simulink model "SistemaUrinarioMasculino"  (R2024b)
settings: Solver=VariableStepAuto  StartTime=0.0  StopTime=30  RelTol=1e-3
libraries: slpidlib x1
settings DataIOCC: ReturnWorkspaceOutputs=off  TimeSaveName=t
settings DebuggingCC: AlgebraicLoopMsg=none  ArtificialAlgebraicLoopMsg=none

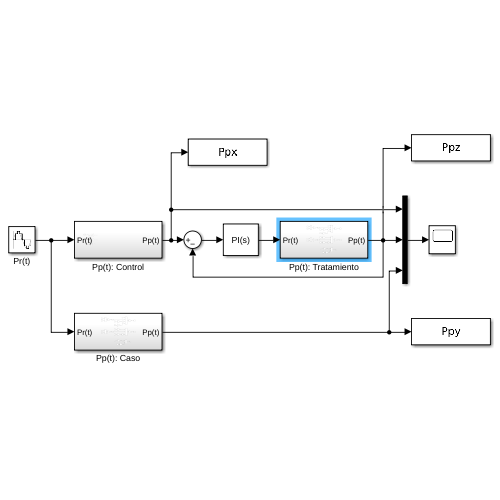
[thumbnail: Simulink's stored preview of the top-level diagram]
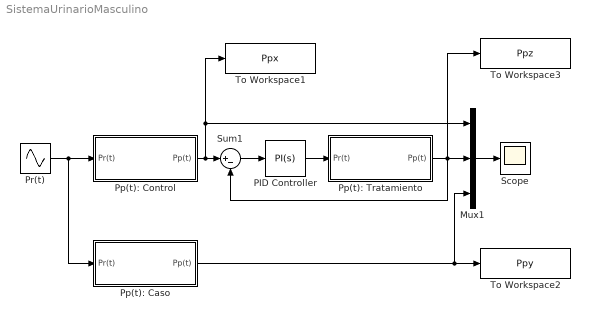
== system SistemaUrinarioMasculino ==
  Mux1 : Mux  Inputs=3
  PID Controller : slpidlib/PID Controller  Controller=PI  Form=Parallel  TimeDomain=Continuous-time  UseExternalTs=off  SampleTime=-1  IntegratorMethod=Forward Euler  FilterMethod=Forward Euler  ControllerParametersSource=internal  P=0.0233322963423837  I=449.984445135772  UseKiTs=off  D=0  UseExternalDerivativeSource=off  N=100  UseFilter=on  TunerSelectOption=Transfer Function Based (PID Tuner App)  InitialConditionSource=internal  InitialConditionForIntegrator=0  InitialConditionForFilter=0  DifferentiatorICPrevScaledInput=0  ExternalReset=none  TrackingMode=off  Kt=1  LimitOutput=off  SatLimitsSource=internal  UpperSaturationLimit=inf  LowerSaturationLimit=-inf  LinearizeAsGain=on  AntiWindupMode=none  Kb=1  LimitIntegrator=off  UpperIntegratorSaturationLimit=inf  LowerIntegratorSaturationLimit=-inf  POutMin=[]  POutMax=[]  IOutMin=[]  IOutMax=[]  DOutMin=[]  DOutMax=[]  NOutMin=[]  NOutMax=[]  SumOutMin=[]  SumOutMax=[]  SaturationOutMin=[]  SaturationOutMax=[]  PParamMin=[]  PParamMax=[]  IParamMin=[]  IParamMax=[]  DParamMin=[]  DParamMax=[]  NParamMin=[]  NParamMax=[]  KbParamMin=[]  KbParamMax=[]  KtParamMin=[]  KtParamMax=[]  KbOutMin=[]  KbOutMax=[]  KtOutMin=[]  KtOutMax=[]  IntegratorOutMin=[]  IntegratorOutMax=[]  FilterOutMin=[]  FilterOutMax=[]  SumI1OutMin=[]  SumI1OutMax=[]  SumI2OutMin=[]  SumI2OutMax=[]  SumI3OutMin=[]  SumI3OutMax=[]  SumI4OutMin=[]  SumI4OutMax=[]  SumDOutMin=[]  SumDOutMax=[]  DifferentiatorOutMin=[]  DifferentiatorOutMax=[]  FilterDiffOutCoefMin=[]  FilterDiffOutCoefMax=[]  ReciprocalOutMin=[]  ReciprocalOutMax=[]  SumDenOutMin=[]  SumDenOutMax=[]  SumNumOutMin=[]  SumNumOutMax=[]  DivideOutMin=[]  DivideOutMax=[]  UdiffTsProdOutMin=[]  UdiffTsProdOutMax=[]  NTsProdOutMin=[]  NTsProdOutMax=[]  UintegralTsProdOutMin=[]  UintegralTsProdOutMax=[]  UngainTsProdOutMin=[]  UngainTsProdOutMax=[]  ClampingZeroOutDataTypeStr=Inherit: Inherit via back propagation  ClampingZeroOutMin=[]  ClampingZeroOutMax=[]  FilterDenConstantOutDataTypeStr=Inherit: Inherit via back propagation  FilterDenConstantOutMin=[]  FilterDenConstantOutMax=[]  PCopyOutDataTypeStr=Inherit: Inherit via back propagation  PCopyOutMin=[]  PCopyOutMax=[]  NCopyOutDataTypeStr=Inherit: Inherit via back propagation  NCopyOutMin=[]  NCopyOutMax=[]  IntegratorContinuousStateAttributes=''  IntegratorStateMustResolveToSignalObject=off  IntegratorRTWStateStorageClass=Auto  FilterContinuousStateAttributes=''  FilterStateMustResolveToSignalObject=off  FilterRTWStateStorageClass=Auto  ParallelPVariant=InternalParameters  IdealPVariant=Disabled  IVariant=InternalParameters  DVariant=Disabled  IntegratorVariant=Continuous  SatVariant=Disabled  AWVariant=Passthrough  PCopyVariant=Disabled  TRVariant=Disabled  FdbkBlocksVariant=Forward  IdealPFdbkVariant=Disabled  SatFdbkVariant=Disabled  DerivativeFilterVariant=Disabled  NVariant=Disabled  NCopyVariant=Disabled_SignalSpec  FilterICVariant=Disabled  IntegratorICVariant=InternalICs  ExternalResetVariant=Disabled  TRSumVariant=Passthrough  SumFdbkVariant=Disabled  SumVariant=Sum_PI  TsampFilterVariant=InternalTs  TsampNgainVariant=Passthrough  TsampIntegralVariant=Disabled_SignalSpec  ExternalSaturationOutDataTypeStr=Inherit: Same as second input  DerivativeSourceVariant=Disabled  PreIntVariant=InternalPreInt
  Pp(t): Caso : Subsystem
  Pp(t): Control : Subsystem
  Pp(t): Tratamiento : Subsystem
  Pr(t) : Sin  Frequency=1.5708  SampleTime=0.001
  Scope : Scope
  Sum1 : Sum  Inputs=|+-
  To Workspace1 : ToWorkspace  VariableName=Ppx  SampleTime=-1
  To Workspace2 : ToWorkspace  VariableName=Ppy  SampleTime=-1
  To Workspace3 : ToWorkspace  VariableName=Ppz  SampleTime=-1
  wires:
  Pr(t)/1 -> Pp(t): Caso/1(Pr(t)), Pp(t): Control/1(Pr(t))
  Pp(t): Control/1(Pp(t)) -> Mux1/1, To Workspace1/1, Sum1/1
  Sum1/1 -> PID Controller/1
  Pp(t): Caso/1(Pp(t)) -> Mux1/3, To Workspace2/1
  PID Controller/1 -> Pp(t): Tratamiento/1(Pr(t))
  Pp(t): Tratamiento/1(Pp(t)) -> Sum1/2, To Workspace3/1, Mux1/2
  Mux1/1 -> Scope/1

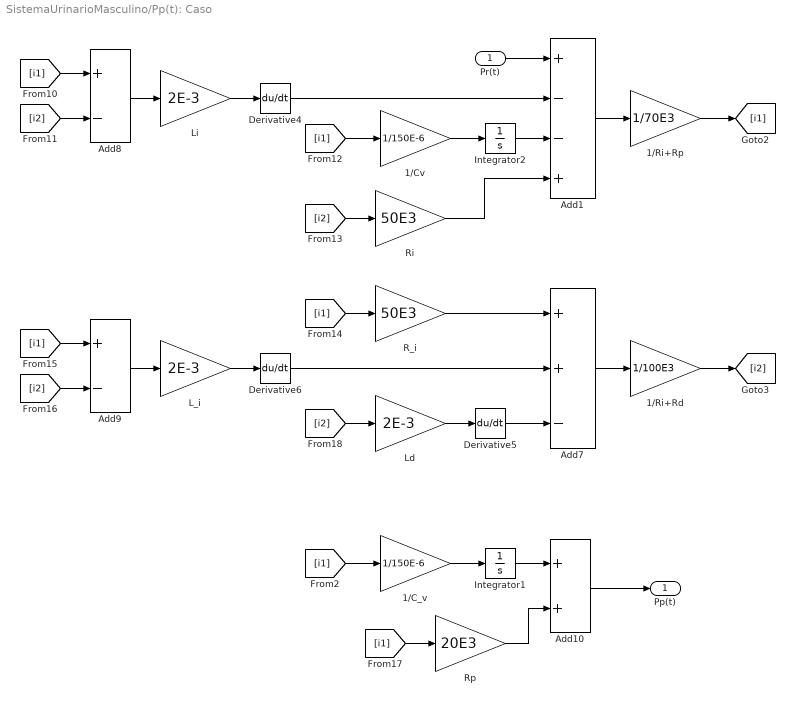
== system SistemaUrinarioMasculino/Pp(t): Caso ==
  Pr(t) : Inport
  1/C_v : Gain  Gain=1/150E-6
  1/Cv : Gain  Gain=1/150E-6
  1/Ri+Rd : Gain  Gain=1/100E3
  1/Ri+Rp : Gain  Gain=1/70E3
  Add1 : Sum  Inputs=+--+
  Add10 : Sum
  Add7 : Sum  Inputs=++-
  Add8 : Sum  Inputs=+-
  Add9 : Sum  Inputs=+-
  Derivative4 : Derivative
  Derivative5 : Derivative
  Derivative6 : Derivative
  Integrator1 : Integrator
  Integrator2 : Integrator
  L_i : Gain  Gain=2E-3
  Ld : Gain  Gain=2E-3
  Li : Gain  Gain=2E-3
  R_i : Gain  Gain=50E3
  Ri : Gain  Gain=50E3
  Rp : Gain  Gain=20E3
  Pp(t) : Outport
  wires:
  Ri/1 -> Add1/4
  Li/1 -> Derivative4/1
  [i2] -> Ld/1
  Add1/1 -> 1/Ri+Rp/1
  Add7/1 -> 1/Ri+Rd/1
  Derivative4/1 -> Add1/2
  [i1] -> 1/Cv/1
  1/Cv/1 -> Integrator2/1
  Add9/1 -> L_i/1
  [i2] -> Ri/1
  Derivative6/1 -> Add7/2
  [i1] -> R_i/1
  Rp/1 -> Add10/2
  Ld/1 -> Derivative5/1
  Add8/1 -> Li/1
  1/Ri+Rp/1 -> [i1]
  [i1] -> Add9/1
  [i2] -> Add9/2
  [i1] -> Rp/1
  1/Ri+Rd/1 -> [i2]
  [i1] -> Add8/1
  Derivative5/1 -> Add7/3
  Integrator2/1 -> Add1/3
  L_i/1 -> Derivative6/1
  Add10/1 -> Pp(t)/1
  Pr(t)/1 -> Add1/1
  R_i/1 -> Add7/1
  [i2] -> Add8/2
  Integrator1/1 -> Add10/1
  [i1] -> 1/C_v/1
  1/C_v/1 -> Integrator1/1

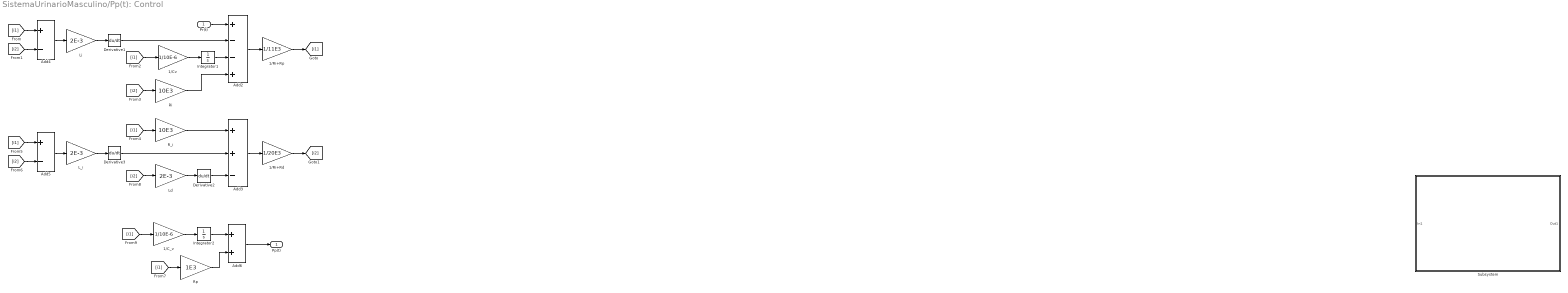
== system SistemaUrinarioMasculino/Pp(t): Control ==
  Pr(t) : Inport
  1/C_v : Gain  Gain=1/10E-6
  1/Cv : Gain  Gain=1/10E-6
  1/Ri+Rd : Gain  Gain=1/20E3
  1/Ri+Rp : Gain  Gain=1/11E3
  Add2 : Sum  Inputs=+--+
  Add3 : Sum  Inputs=++-
  Add4 : Sum  Inputs=+-
  Add5 : Sum  Inputs=+-
  Add6 : Sum
  Derivative1 : Derivative
  Derivative2 : Derivative
  Derivative3 : Derivative
  Integrator1 : Integrator
  Integrator2 : Integrator
  L_i : Gain  Gain=2E-3
  Ld : Gain  Gain=2E-3
  Li : Gain  Gain=2E-3
  R_i : Gain  Gain=10E3
  Ri : Gain  Gain=10E3
  Rp : Gain  Gain=1E3
  Subsystem : Subsystem
  Pp(t) : Outport
  wires:
  Pr(t)/1 -> Add2/1
  Add2/1 -> 1/Ri+Rp/1
  Add4/1 -> Li/1
  Derivative1/1 -> Add2/2
  Li/1 -> Derivative1/1
  Integrator1/1 -> Add2/3
  [i1] -> Add4/1
  [i2] -> Add4/2
  1/Ri+Rp/1 -> [i1]
  1/Cv/1 -> Integrator1/1
  [i1] -> 1/Cv/1
  Ri/1 -> Add2/4
  [i2] -> Ri/1
  [i1] -> R_i/1
  Add3/1 -> 1/Ri+Rd/1
  1/Ri+Rd/1 -> [i2]
  [i1] -> Add5/1
  Add5/1 -> L_i/1
  L_i/1 -> Derivative3/1
  [i2] -> Add5/2
  Derivative3/1 -> Add3/2
  Ld/1 -> Derivative2/1
  R_i/1 -> Add3/1
  [i2] -> Ld/1
  Derivative2/1 -> Add3/3
  Rp/1 -> Add6/2
  [i1] -> Rp/1
  Add6/1 -> Pp(t)/1
  [i1] -> 1/C_v/1
  1/C_v/1 -> Integrator2/1
  Integrator2/1 -> Add6/1

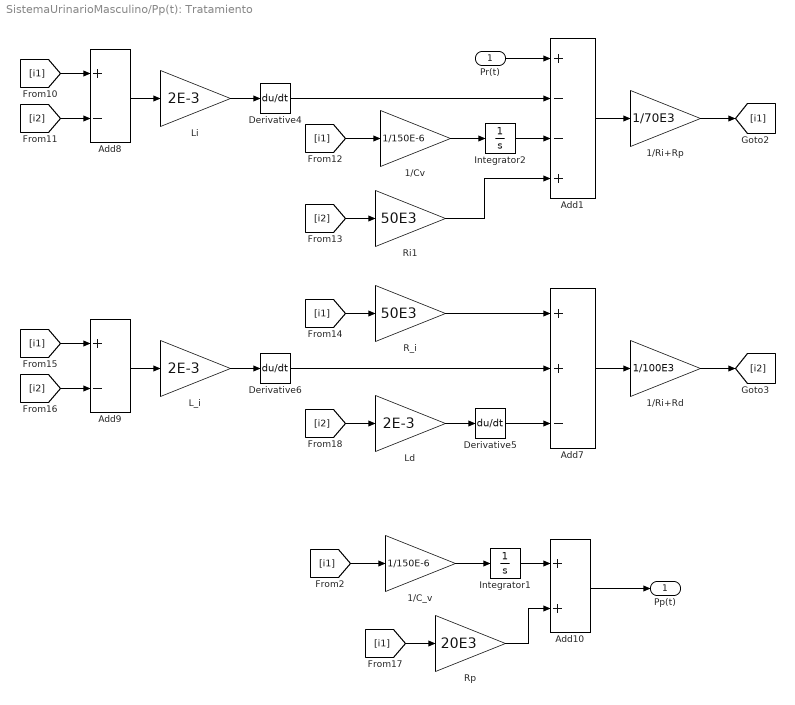
== system SistemaUrinarioMasculino/Pp(t): Tratamiento ==
  Pr(t) : Inport
  1/C_v : Gain  Gain=1/150E-6
  1/Cv : Gain  Gain=1/150E-6
  1/Ri+Rd : Gain  Gain=1/100E3
  1/Ri+Rp : Gain  Gain=1/70E3
  Add1 : Sum  Inputs=+--+
  Add10 : Sum
  Add7 : Sum  Inputs=++-
  Add8 : Sum  Inputs=+-
  Add9 : Sum  Inputs=+-
  Derivative4 : Derivative
  Derivative5 : Derivative
  Derivative6 : Derivative
  Integrator1 : Integrator
  Integrator2 : Integrator
  L_i : Gain  Gain=2E-3
  Ld : Gain  Gain=2E-3
  Li : Gain  Gain=2E-3
  R_i : Gain  Gain=50E3
  Ri1 : Gain  Gain=50E3
  Rp : Gain  Gain=20E3
  Pp(t) : Outport
  wires:
  Add10/1 -> Pp(t)/1
  Add7/1 -> 1/Ri+Rd/1
  R_i/1 -> Add7/1
  [i1] -> Rp/1
  Derivative5/1 -> Add7/3
  Ld/1 -> Derivative5/1
  Li/1 -> Derivative4/1
  Derivative4/1 -> Add1/2
  L_i/1 -> Derivative6/1
  Derivative6/1 -> Add7/2
  Rp/1 -> Add10/2
  [i1] -> Add9/1
  [i2] -> Ld/1
  Integrator2/1 -> Add1/3
  Add9/1 -> L_i/1
  Ri1/1 -> Add1/4
  [i2] -> Add9/2
  [i2] -> Add8/2
  [i1] -> Add8/1
  [i2] -> Ri1/1
  1/Cv/1 -> Integrator2/1
  1/Ri+Rp/1 -> [i1]
  [i1] -> R_i/1
  Add1/1 -> 1/Ri+Rp/1
  Add8/1 -> Li/1
  [i1] -> 1/Cv/1
  Pr(t)/1 -> Add1/1
  1/Ri+Rd/1 -> [i2]
  Integrator1/1 -> Add10/1
  [i1] -> 1/C_v/1
  1/C_v/1 -> Integrator1/1

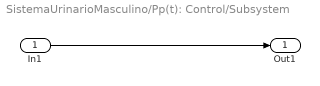
== system SistemaUrinarioMasculino/Pp(t): Control/Subsystem ==
  In1 : Inport
  Out1 : Outport
  wires:
  In1/1 -> Out1/1
